simulink subsystem "convertRawGyro"  (R2024a)
settings: Solver=VariableStepAuto  StartTime=0.0  StopTime=10.0  RelTol=1e-3
libraries: hdlsllib x3, simulink x3
settings Model: Creator=Peter  LastModifiedBy=Peter

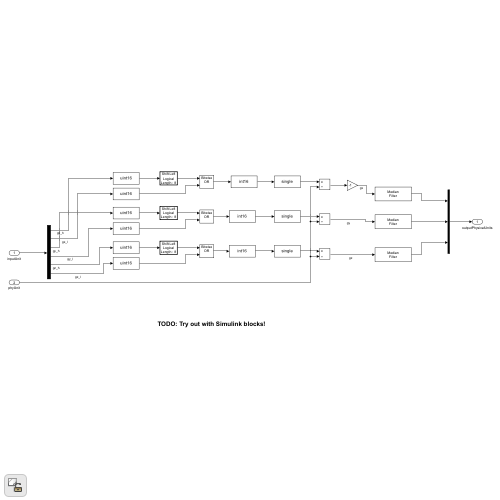
[thumbnail: Simulink's stored preview of the top-level diagram]
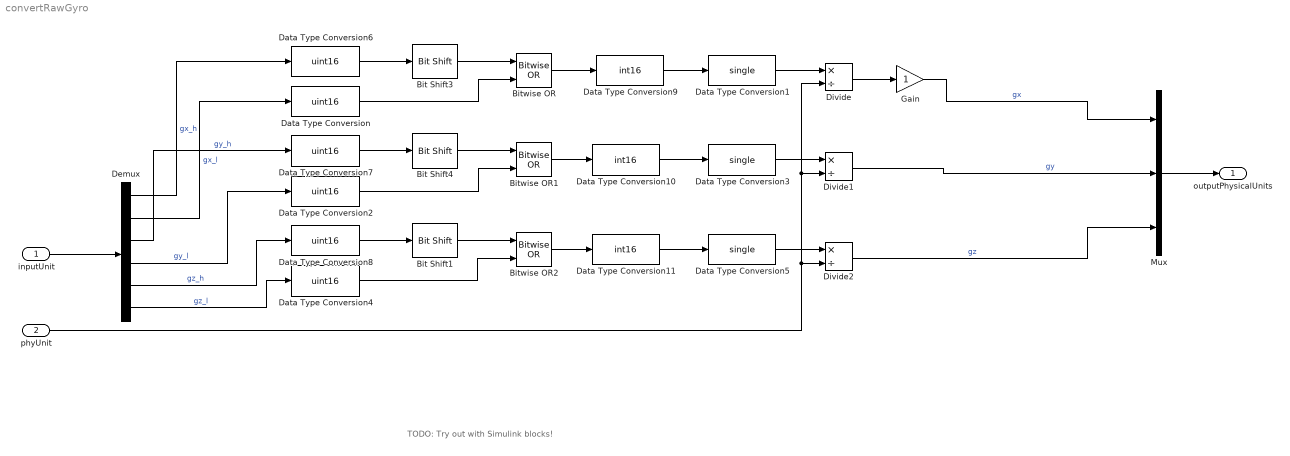
== system convertRawGyro ==
  note: TODO: Try out with Simulink blocks!
  inputUnit : Inport
  phyUnit : Inport  Port=2
  Bit Shift1 : hdlsllib/Logic and Bit Operations/Bit Shift  mode=Shift Left Logical  N=8
  Bit Shift3 : hdlsllib/Logic and Bit Operations/Bit Shift  mode=Shift Left Logical  N=8
  Bit Shift4 : hdlsllib/Logic and Bit Operations/Bit Shift  mode=Shift Left Logical  N=8
  Bitwise OR : simulink/Logic and Bit Operations/Bitwise Operator  logicop=OR  UseBitMask=off  NumInputPorts=2  BitMask=bin2dec('11011001')  BitMaskRealWorld=Stored Integer
      settings: LibrarySourceBlock=|
      | simulink/Quick Insert/Logic and Bit
      | Operations/Bitwise OR
  Bitwise OR1 : simulink/Logic and Bit Operations/Bitwise Operator  logicop=OR  UseBitMask=off  NumInputPorts=2  BitMask=bin2dec('11011001')  BitMaskRealWorld=Stored Integer
      settings: LibrarySourceBlock=|
      | simulink/Quick Insert/Logic and Bit
      | Operations/Bitwise OR
  Bitwise OR2 : simulink/Logic and Bit Operations/Bitwise Operator  logicop=OR  UseBitMask=off  NumInputPorts=2  BitMask=bin2dec('11011001')  BitMaskRealWorld=Stored Integer
      settings: LibrarySourceBlock=|
      | simulink/Quick Insert/Logic and Bit
      | Operations/Bitwise OR
  Data Type Conversion{,2,4,6..8} (6 alike) : DataTypeConversion  OutDataTypeStr=uint16  SaturateOnIntegerOverflow=off  RndMeth=Floor
  Data Type Conversion1 : DataTypeConversion  OutDataTypeStr=single  SaturateOnIntegerOverflow=off  RndMeth=Floor
  Data Type Conversion10 : DataTypeConversion  OutDataTypeStr=int16  SaturateOnIntegerOverflow=off  RndMeth=Floor
  Data Type Conversion11 : DataTypeConversion  OutDataTypeStr=int16  SaturateOnIntegerOverflow=off  RndMeth=Floor
  Data Type Conversion3 : DataTypeConversion  OutDataTypeStr=single  SaturateOnIntegerOverflow=off  RndMeth=Floor
  Data Type Conversion5 : DataTypeConversion  OutDataTypeStr=single  SaturateOnIntegerOverflow=off  RndMeth=Floor
  Data Type Conversion9 : DataTypeConversion  OutDataTypeStr=int16  SaturateOnIntegerOverflow=off  RndMeth=Floor
  Demux : Demux  Outputs=6
  Divide : Product  Inputs=*/
  Divide1 : Product  Inputs=*/
  Divide2 : Product  Inputs=*/
  Gain : Gain
  Mux : Mux  Inputs=3
  outputPhysicalUnits : Outport
  wires:
  inputUnit/1 -> Demux/1
  Demux/1 -> Data Type Conversion6/1  "gx_h"
  Demux/2 -> Data Type Conversion/1  "gx_l"
  Data Type Conversion/1 -> Bitwise OR/2
  Bitwise OR/1 -> Data Type Conversion9/1
  Data Type Conversion1/1 -> Divide/1
  Data Type Conversion3/1 -> Divide1/1
  Bitwise OR1/1 -> Data Type Conversion10/1
  Data Type Conversion2/1 -> Bitwise OR1/2
  Demux/4 -> Data Type Conversion2/1  "gy_l"
  Demux/3 -> Data Type Conversion7/1  "gy_h"
  Demux/5 -> Data Type Conversion8/1  "gz_h"
  Demux/6 -> Data Type Conversion4/1  "gz_l"
  Data Type Conversion4/1 -> Bitwise OR2/2
  Bitwise OR2/1 -> Data Type Conversion11/1
  Data Type Conversion5/1 -> Divide2/1
  Divide/1 -> Gain/1
  Divide2/1 -> Mux/3  "gz"
  Divide1/1 -> Mux/2  "gy"
  phyUnit/1 -> Divide2/2, Divide1/2, Divide/2
  Gain/1 -> Mux/1  "gx"
  Mux/1 -> outputPhysicalUnits/1
  Data Type Conversion6/1 -> Bit Shift3/1
  Data Type Conversion7/1 -> Bit Shift4/1
  Data Type Conversion8/1 -> Bit Shift1/1
  Data Type Conversion9/1 -> Data Type Conversion1/1
  Data Type Conversion10/1 -> Data Type Conversion3/1
  Data Type Conversion11/1 -> Data Type Conversion5/1
  Bit Shift3/1 -> Bitwise OR/1
  Bit Shift4/1 -> Bitwise OR1/1
  Bit Shift1/1 -> Bitwise OR2/1
